simulink model "Ieee14_CC_2019b"  (R2019b)
settings: Solver=ode1  StartTime=0.0  StopTime=3600  FixedStep=1e-3  MaxStep=1e-4  RelTol=1e-3
model workspace (MAT data in the model file):
  pruebaValor = 0
libraries: powerlib x118, dspnetwork x116, source_mod x14, simulink x1
(part 3 of 3)

== system Ieee14_CC_2019b/SM 2 ==
  Constant : Constant  Value=0
  Constant1 : Constant
  Constant2 : Constant  Value=2
  Constant3 : Constant  Value=0
  Constant4 : Constant
  Constant5 : Constant  Value=2
  Index Vector{,1..5} (6 alike) : MultiPortSwitch  DataPortOrder=Zero-based contiguous  Inputs=1  zeroidx=on
  Three-Phase V-I Measurement : powerlib/Measurements/Three-Phase V-I Measurement  VoltageMeasurement=phase-to-ground  SetLabelV=off  LabelV=Vabc  Vpu=on  VpuLL=off  CurrentMeasurement=yes  SetLabelI=off  LabelI=Iabc  Ipu=on  Pbase=100e6  Vbase=69e3  OutputType=Complex  PhasorSimulation=off  PSBequivalent=0
      settings: SourceProductName=Simscape Electrical
  UDP Send Ia : dspnetwork/UDP Send  remoteURL='10.0.255.255'  remotePort=20022  localURL='255.255.255.255'  localPortSource=Automatically determine  localPort=-1  sampletime=-1  blockPlatform=LINUX  separateLengthPort=0
      settings: SourceProductName=Simulink
  UDP Send Ib : dspnetwork/UDP Send  remoteURL='10.0.255.255'  remotePort=20021  localURL='255.255.255.255'  localPortSource=Automatically determine  localPort=-1  sampletime=-1  blockPlatform=LINUX  separateLengthPort=0
      settings: SourceProductName=Simulink
  UDP Send Ic : dspnetwork/UDP Send  remoteURL='10.0.255.255'  remotePort=20020  localURL='255.255.255.255'  localPortSource=Automatically determine  localPort=-1  sampletime=-1  blockPlatform=LINUX  separateLengthPort=0
      settings: SourceProductName=Simulink
  UDP Send Va : dspnetwork/UDP Send  remoteURL='10.0.255.255'  remotePort=10020  localURL='255.255.255.255'  localPortSource=Automatically determine  localPort=-1  sampletime=-1  blockPlatform=LINUX  separateLengthPort=0
      settings: SourceProductName=Simulink
  UDP Send Vb : dspnetwork/UDP Send  remoteURL='10.0.255.255'  remotePort=10021  localURL='255.255.255.255'  localPortSource=Automatically determine  localPort=-1  sampletime=-1  blockPlatform=LINUX  separateLengthPort=0
      settings: SourceProductName=Simulink
  UDP Send Vc : dspnetwork/UDP Send  remoteURL='10.0.255.255'  remotePort=10022  localURL='255.255.255.255'  localPortSource=Automatically determine  localPort=-1  sampletime=-1  blockPlatform=LINUX  separateLengthPort=0
      settings: SourceProductName=Simulink
  a : PMIOPort  Side=Left
  b : PMIOPort  Port=2  Side=Left
  c : PMIOPort  Port=3  Side=Left
  A : PMIOPort  Port=4  Side=Right
  B : PMIOPort  Port=5  Side=Right
  C : PMIOPort  Port=6  Side=Right
  Vabc : Outport
  Iabc : Outport  Port=2
  wires:
  Index Vector/1 -> UDP Send Va/1
  Constant1/1 -> Index Vector1/1
  Constant/1 -> Index Vector/1
  Index Vector2/1 -> UDP Send Vc/1
  Index Vector1/1 -> UDP Send Vb/1
  Constant2/1 -> Index Vector2/1
  Three-Phase V-I Measurement/1 -> Index Vector2/2, Index Vector/2, Index Vector1/2, Vabc/1
  Index Vector4/1 -> UDP Send Ib/1
  Constant3/1 -> Index Vector3/1
  Index Vector3/1 -> UDP Send Ic/1
  Constant5/1 -> Index Vector5/1
  Constant4/1 -> Index Vector4/1
  Index Vector5/1 -> UDP Send Ia/1
  Three-Phase V-I Measurement/2 -> Iabc/1, Index Vector3/2, Index Vector4/2, Index Vector5/2
  connections:
  b/RConn1 -- Three-Phase V-I Measurement/RConn2
  a/RConn1 -- Three-Phase V-I Measurement/RConn1
  c/RConn1 -- Three-Phase V-I Measurement/RConn3
  A/RConn1 -- Three-Phase V-I Measurement/LConn1
  B/RConn1 -- Three-Phase V-I Measurement/LConn2
  C/RConn1 -- Three-Phase V-I Measurement/LConn3

== system Ieee14_CC_2019b/SM 3 ==
  Constant : Constant  Value=0
  Constant1 : Constant
  Constant2 : Constant  Value=2
  Constant3 : Constant  Value=0
  Constant4 : Constant
  Constant5 : Constant  Value=2
  Index Vector{,1..5} (6 alike) : MultiPortSwitch  DataPortOrder=Zero-based contiguous  Inputs=1  zeroidx=on
  Three-Phase V-I Measurement : powerlib/Measurements/Three-Phase V-I Measurement  VoltageMeasurement=phase-to-ground  SetLabelV=off  LabelV=Vabc  Vpu=on  VpuLL=off  CurrentMeasurement=yes  SetLabelI=off  LabelI=Iabc  Ipu=on  Pbase=100e6  Vbase=69e3  OutputType=Complex  PhasorSimulation=off  PSBequivalent=0
      settings: SourceProductName=Simscape Electrical
  UDP Send Ia : dspnetwork/UDP Send  remoteURL='10.0.255.255'  remotePort=20032  localURL='255.255.255.255'  localPortSource=Automatically determine  localPort=-1  sampletime=-1  blockPlatform=LINUX  separateLengthPort=0
      settings: SourceProductName=Simulink
  UDP Send Ib : dspnetwork/UDP Send  remoteURL='10.0.255.255'  remotePort=20031  localURL='255.255.255.255'  localPortSource=Automatically determine  localPort=-1  sampletime=-1  blockPlatform=LINUX  separateLengthPort=0
      settings: SourceProductName=Simulink
  UDP Send Ic : dspnetwork/UDP Send  remoteURL='10.0.255.255'  remotePort=20030  localURL='255.255.255.255'  localPortSource=Automatically determine  localPort=-1  sampletime=-1  blockPlatform=LINUX  separateLengthPort=0
      settings: SourceProductName=Simulink
  UDP Send Va : dspnetwork/UDP Send  remoteURL='10.0.255.255'  remotePort=10030  localURL='255.255.255.255'  localPortSource=Automatically determine  localPort=-1  sampletime=-1  blockPlatform=LINUX  separateLengthPort=0
      settings: SourceProductName=Simulink
  UDP Send Vb : dspnetwork/UDP Send  remoteURL='10.0.255.255'  remotePort=10031  localURL='255.255.255.255'  localPortSource=Automatically determine  localPort=-1  sampletime=-1  blockPlatform=LINUX  separateLengthPort=0
      settings: SourceProductName=Simulink
  UDP Send Vc : dspnetwork/UDP Send  remoteURL='10.0.255.255'  remotePort=10032  localURL='255.255.255.255'  localPortSource=Automatically determine  localPort=-1  sampletime=-1  blockPlatform=LINUX  separateLengthPort=0
      settings: SourceProductName=Simulink
  a : PMIOPort  Side=Left
  b : PMIOPort  Port=2  Side=Left
  c : PMIOPort  Port=3  Side=Left
  A : PMIOPort  Port=4  Side=Right
  B : PMIOPort  Port=5  Side=Right
  C : PMIOPort  Port=6  Side=Right
  Vabc : Outport
  Iabc : Outport  Port=2
  wires:
  Index Vector/1 -> UDP Send Va/1
  Constant1/1 -> Index Vector1/1
  Constant/1 -> Index Vector/1
  Index Vector2/1 -> UDP Send Vc/1
  Index Vector1/1 -> UDP Send Vb/1
  Constant2/1 -> Index Vector2/1
  Three-Phase V-I Measurement/1 -> Index Vector2/2, Index Vector/2, Index Vector1/2, Vabc/1
  Index Vector4/1 -> UDP Send Ib/1
  Constant3/1 -> Index Vector3/1
  Index Vector3/1 -> UDP Send Ic/1
  Constant5/1 -> Index Vector5/1
  Constant4/1 -> Index Vector4/1
  Index Vector5/1 -> UDP Send Ia/1
  Three-Phase V-I Measurement/2 -> Iabc/1, Index Vector3/2, Index Vector4/2, Index Vector5/2
  connections:
  b/RConn1 -- Three-Phase V-I Measurement/RConn2
  a/RConn1 -- Three-Phase V-I Measurement/RConn1
  c/RConn1 -- Three-Phase V-I Measurement/RConn3
  A/RConn1 -- Three-Phase V-I Measurement/LConn1
  B/RConn1 -- Three-Phase V-I Measurement/LConn2
  C/RConn1 -- Three-Phase V-I Measurement/LConn3

== system Ieee14_CC_2019b/SM 4 ==
  Constant : Constant  Value=0
  Constant1 : Constant
  Constant2 : Constant  Value=2
  Constant3 : Constant  Value=0
  Constant4 : Constant
  Constant5 : Constant  Value=2
  Index Vector{,1..5} (6 alike) : MultiPortSwitch  DataPortOrder=Zero-based contiguous  Inputs=1  zeroidx=on
  Three-Phase V-I Measurement : powerlib/Measurements/Three-Phase V-I Measurement  VoltageMeasurement=phase-to-ground  SetLabelV=off  LabelV=Vabc  Vpu=on  VpuLL=off  CurrentMeasurement=yes  SetLabelI=off  LabelI=Iabc  Ipu=on  Pbase=100e6  Vbase=69e3  OutputType=Complex  PhasorSimulation=off  PSBequivalent=0
      settings: SourceProductName=Simscape Electrical
  UDP Send Ia : dspnetwork/UDP Send  remoteURL='10.0.255.255'  remotePort=20042  localURL='255.255.255.255'  localPortSource=Automatically determine  localPort=-1  sampletime=-1  blockPlatform=LINUX  separateLengthPort=0
      settings: SourceProductName=Simulink
  UDP Send Ib : dspnetwork/UDP Send  remoteURL='10.0.255.255'  remotePort=20041  localURL='255.255.255.255'  localPortSource=Automatically determine  localPort=-1  sampletime=-1  blockPlatform=LINUX  separateLengthPort=0
      settings: SourceProductName=Simulink
  UDP Send Ic : dspnetwork/UDP Send  remoteURL='10.0.255.255'  remotePort=20040  localURL='255.255.255.255'  localPortSource=Automatically determine  localPort=-1  sampletime=-1  blockPlatform=LINUX  separateLengthPort=0
      settings: SourceProductName=Simulink
  UDP Send Va : dspnetwork/UDP Send  remoteURL='10.0.255.255'  remotePort=10040  localURL='255.255.255.255'  localPortSource=Automatically determine  localPort=-1  sampletime=-1  blockPlatform=LINUX  separateLengthPort=0
      settings: SourceProductName=Simulink
  UDP Send Vb : dspnetwork/UDP Send  remoteURL='10.0.255.255'  remotePort=10041  localURL='255.255.255.255'  localPortSource=Automatically determine  localPort=-1  sampletime=-1  blockPlatform=LINUX  separateLengthPort=0
      settings: SourceProductName=Simulink
  UDP Send Vc : dspnetwork/UDP Send  remoteURL='10.0.255.255'  remotePort=10042  localURL='255.255.255.255'  localPortSource=Automatically determine  localPort=-1  sampletime=-1  blockPlatform=LINUX  separateLengthPort=0
      settings: SourceProductName=Simulink
  a : PMIOPort  Side=Left
  b : PMIOPort  Port=2  Side=Left
  c : PMIOPort  Port=3  Side=Left
  A : PMIOPort  Port=4  Side=Right
  B : PMIOPort  Port=5  Side=Right
  C : PMIOPort  Port=6  Side=Right
  Vabc : Outport
  Iabc : Outport  Port=2
  wires:
  Index Vector/1 -> UDP Send Va/1
  Constant1/1 -> Index Vector1/1
  Constant/1 -> Index Vector/1
  Index Vector2/1 -> UDP Send Vc/1
  Index Vector1/1 -> UDP Send Vb/1
  Constant2/1 -> Index Vector2/1
  Three-Phase V-I Measurement/1 -> Index Vector2/2, Index Vector/2, Index Vector1/2, Vabc/1
  Index Vector4/1 -> UDP Send Ib/1
  Constant3/1 -> Index Vector3/1
  Index Vector3/1 -> UDP Send Ic/1
  Constant5/1 -> Index Vector5/1
  Constant4/1 -> Index Vector4/1
  Index Vector5/1 -> UDP Send Ia/1
  Three-Phase V-I Measurement/2 -> Iabc/1, Index Vector3/2, Index Vector4/2, Index Vector5/2
  connections:
  b/RConn1 -- Three-Phase V-I Measurement/RConn2
  a/RConn1 -- Three-Phase V-I Measurement/RConn1
  c/RConn1 -- Three-Phase V-I Measurement/RConn3
  A/RConn1 -- Three-Phase V-I Measurement/LConn1
  B/RConn1 -- Three-Phase V-I Measurement/LConn2
  C/RConn1 -- Three-Phase V-I Measurement/LConn3

== system Ieee14_CC_2019b/SM 5 ==
  Constant : Constant  Value=0
  Constant1 : Constant
  Constant2 : Constant  Value=2
  Constant3 : Constant  Value=0
  Constant4 : Constant
  Constant5 : Constant  Value=2
  Index Vector{,1..5} (6 alike) : MultiPortSwitch  DataPortOrder=Zero-based contiguous  Inputs=1  zeroidx=on
  Three-Phase V-I Measurement : powerlib/Measurements/Three-Phase V-I Measurement  VoltageMeasurement=phase-to-ground  SetLabelV=off  LabelV=Vabc  Vpu=on  VpuLL=off  CurrentMeasurement=yes  SetLabelI=off  LabelI=Iabc  Ipu=on  Pbase=100e6  Vbase=69e3  OutputType=Complex  PhasorSimulation=off  PSBequivalent=0
      settings: SourceProductName=Simscape Electrical
  UDP Send Ia : dspnetwork/UDP Send  remoteURL='10.0.255.255'  remotePort=20052  localURL='255.255.255.255'  localPortSource=Automatically determine  localPort=-1  sampletime=-1  blockPlatform=LINUX  separateLengthPort=0
      settings: SourceProductName=Simulink
  UDP Send Ib : dspnetwork/UDP Send  remoteURL='10.0.255.255'  remotePort=20051  localURL='255.255.255.255'  localPortSource=Automatically determine  localPort=-1  sampletime=-1  blockPlatform=LINUX  separateLengthPort=0
      settings: SourceProductName=Simulink
  UDP Send Ic : dspnetwork/UDP Send  remoteURL='10.0.255.255'  remotePort=20050  localURL='255.255.255.255'  localPortSource=Automatically determine  localPort=-1  sampletime=-1  blockPlatform=LINUX  separateLengthPort=0
      settings: SourceProductName=Simulink
  UDP Send Va : dspnetwork/UDP Send  remoteURL='10.0.255.255'  remotePort=10050  localURL='255.255.255.255'  localPortSource=Automatically determine  localPort=-1  sampletime=-1  blockPlatform=LINUX  separateLengthPort=0
      settings: SourceProductName=Simulink
  UDP Send Vb : dspnetwork/UDP Send  remoteURL='10.0.255.255'  remotePort=10051  localURL='255.255.255.255'  localPortSource=Automatically determine  localPort=-1  sampletime=-1  blockPlatform=LINUX  separateLengthPort=0
      settings: SourceProductName=Simulink
  UDP Send Vc : dspnetwork/UDP Send  remoteURL='10.0.255.255'  remotePort=10052  localURL='255.255.255.255'  localPortSource=Automatically determine  localPort=-1  sampletime=-1  blockPlatform=LINUX  separateLengthPort=0
      settings: SourceProductName=Simulink
  a : PMIOPort  Side=Left
  b : PMIOPort  Port=2  Side=Left
  c : PMIOPort  Port=3  Side=Left
  A : PMIOPort  Port=4  Side=Right
  B : PMIOPort  Port=5  Side=Right
  C : PMIOPort  Port=6  Side=Right
  Vabc : Outport
  Iabc : Outport  Port=2
  wires:
  Index Vector/1 -> UDP Send Va/1
  Constant1/1 -> Index Vector1/1
  Constant/1 -> Index Vector/1
  Index Vector2/1 -> UDP Send Vc/1
  Index Vector1/1 -> UDP Send Vb/1
  Constant2/1 -> Index Vector2/1
  Three-Phase V-I Measurement/1 -> Index Vector2/2, Index Vector/2, Index Vector1/2, Vabc/1
  Index Vector4/1 -> UDP Send Ib/1
  Constant3/1 -> Index Vector3/1
  Index Vector3/1 -> UDP Send Ic/1
  Constant5/1 -> Index Vector5/1
  Constant4/1 -> Index Vector4/1
  Index Vector5/1 -> UDP Send Ia/1
  Three-Phase V-I Measurement/2 -> Iabc/1, Index Vector3/2, Index Vector4/2, Index Vector5/2
  connections:
  b/RConn1 -- Three-Phase V-I Measurement/RConn2
  a/RConn1 -- Three-Phase V-I Measurement/RConn1
  c/RConn1 -- Three-Phase V-I Measurement/RConn3
  A/RConn1 -- Three-Phase V-I Measurement/LConn1
  B/RConn1 -- Three-Phase V-I Measurement/LConn2
  C/RConn1 -- Three-Phase V-I Measurement/LConn3

== system Ieee14_CC_2019b/SM 6 ==
  Constant : Constant  Value=0
  Constant1 : Constant
  Constant2 : Constant  Value=2
  Constant3 : Constant  Value=0
  Constant4 : Constant
  Constant5 : Constant  Value=2
  Index Vector{,1..5} (6 alike) : MultiPortSwitch  DataPortOrder=Zero-based contiguous  Inputs=1  zeroidx=on
  Three-Phase V-I Measurement : powerlib/Measurements/Three-Phase V-I Measurement  VoltageMeasurement=phase-to-ground  SetLabelV=off  LabelV=Vabc  Vpu=on  VpuLL=off  CurrentMeasurement=yes  SetLabelI=off  LabelI=Iabc  Ipu=on  Pbase=100e6  Vbase=69e3  OutputType=Complex  PhasorSimulation=off  PSBequivalent=0
      settings: SourceProductName=Simscape Electrical
  UDP Send Ia : dspnetwork/UDP Send  remoteURL='10.0.255.255'  remotePort=20062  localURL='255.255.255.255'  localPortSource=Automatically determine  localPort=-1  sampletime=-1  blockPlatform=LINUX  separateLengthPort=0
      settings: SourceProductName=Simulink
  UDP Send Ib : dspnetwork/UDP Send  remoteURL='10.0.255.255'  remotePort=20061  localURL='255.255.255.255'  localPortSource=Automatically determine  localPort=-1  sampletime=-1  blockPlatform=LINUX  separateLengthPort=0
      settings: SourceProductName=Simulink
  UDP Send Ic : dspnetwork/UDP Send  remoteURL='10.0.255.255'  remotePort=20060  localURL='255.255.255.255'  localPortSource=Automatically determine  localPort=-1  sampletime=-1  blockPlatform=LINUX  separateLengthPort=0
      settings: SourceProductName=Simulink
  UDP Send Va : dspnetwork/UDP Send  remoteURL='10.0.255.255'  remotePort=10060  localURL='255.255.255.255'  localPortSource=Automatically determine  localPort=-1  sampletime=-1  blockPlatform=LINUX  separateLengthPort=0
      settings: SourceProductName=Simulink
  UDP Send Vb : dspnetwork/UDP Send  remoteURL='10.0.255.255'  remotePort=10061  localURL='255.255.255.255'  localPortSource=Automatically determine  localPort=-1  sampletime=-1  blockPlatform=LINUX  separateLengthPort=0
      settings: SourceProductName=Simulink
  UDP Send Vc : dspnetwork/UDP Send  remoteURL='10.0.255.255'  remotePort=10062  localURL='255.255.255.255'  localPortSource=Automatically determine  localPort=-1  sampletime=-1  blockPlatform=LINUX  separateLengthPort=0
      settings: SourceProductName=Simulink
  a : PMIOPort  Side=Left
  b : PMIOPort  Port=2  Side=Left
  c : PMIOPort  Port=3  Side=Left
  A : PMIOPort  Port=4  Side=Right
  B : PMIOPort  Port=5  Side=Right
  C : PMIOPort  Port=6  Side=Right
  Vabc : Outport
  Iabc : Outport  Port=2
  wires:
  Index Vector/1 -> UDP Send Va/1
  Constant1/1 -> Index Vector1/1
  Constant/1 -> Index Vector/1
  Index Vector2/1 -> UDP Send Vc/1
  Index Vector1/1 -> UDP Send Vb/1
  Constant2/1 -> Index Vector2/1
  Three-Phase V-I Measurement/1 -> Index Vector2/2, Index Vector/2, Index Vector1/2, Vabc/1
  Index Vector4/1 -> UDP Send Ib/1
  Constant3/1 -> Index Vector3/1
  Index Vector3/1 -> UDP Send Ic/1
  Constant5/1 -> Index Vector5/1
  Constant4/1 -> Index Vector4/1
  Index Vector5/1 -> UDP Send Ia/1
  Three-Phase V-I Measurement/2 -> Iabc/1, Index Vector3/2, Index Vector4/2, Index Vector5/2
  connections:
  b/RConn1 -- Three-Phase V-I Measurement/RConn2
  a/RConn1 -- Three-Phase V-I Measurement/RConn1
  c/RConn1 -- Three-Phase V-I Measurement/RConn3
  A/RConn1 -- Three-Phase V-I Measurement/LConn1
  B/RConn1 -- Three-Phase V-I Measurement/LConn2
  C/RConn1 -- Three-Phase V-I Measurement/LConn3

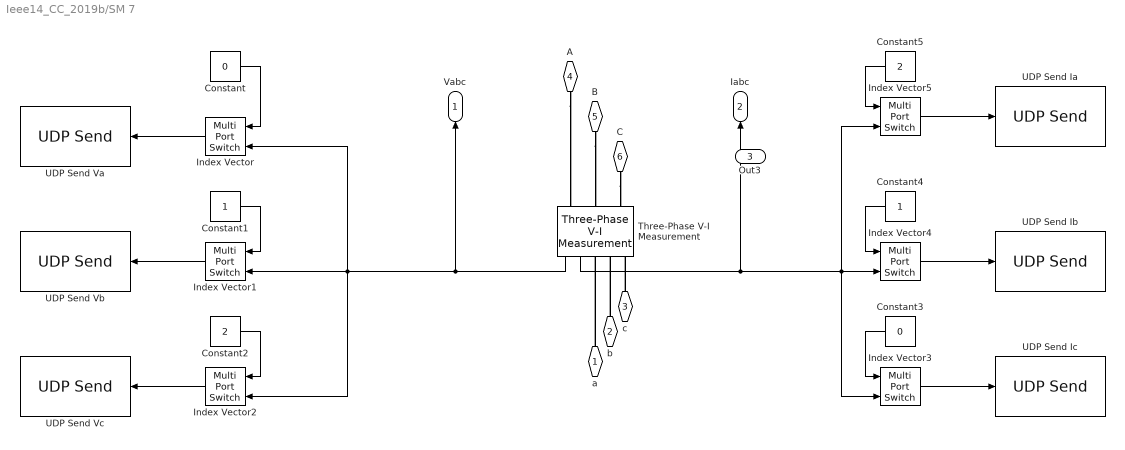
== system Ieee14_CC_2019b/SM 7 ==
  Constant : Constant  Value=0
  Constant1 : Constant
  Constant2 : Constant  Value=2
  Constant3 : Constant  Value=0
  Constant4 : Constant
  Constant5 : Constant  Value=2
  Index Vector{,1..5} (6 alike) : MultiPortSwitch  DataPortOrder=Zero-based contiguous  Inputs=1  zeroidx=on
  Three-Phase V-I Measurement : powerlib/Measurements/Three-Phase V-I Measurement  VoltageMeasurement=phase-to-ground  SetLabelV=off  LabelV=Vabc  Vpu=on  VpuLL=off  CurrentMeasurement=yes  SetLabelI=off  LabelI=Iabc  Ipu=on  Pbase=100e6  Vbase=69e3  OutputType=Complex  PhasorSimulation=off  PSBequivalent=0
      settings: SourceProductName=Simscape Electrical
  UDP Send Ia : dspnetwork/UDP Send  remoteURL='10.0.255.255'  remotePort=20072  localURL='255.255.255.255'  localPortSource=Automatically determine  localPort=-1  sampletime=-1  blockPlatform=LINUX  separateLengthPort=0
      settings: SourceProductName=Simulink
  UDP Send Ib : dspnetwork/UDP Send  remoteURL='10.0.255.255'  remotePort=20071  localURL='255.255.255.255'  localPortSource=Automatically determine  localPort=-1  sampletime=-1  blockPlatform=LINUX  separateLengthPort=0
      settings: SourceProductName=Simulink
  UDP Send Ic : dspnetwork/UDP Send  remoteURL='10.0.255.255'  remotePort=20070  localURL='255.255.255.255'  localPortSource=Automatically determine  localPort=-1  sampletime=-1  blockPlatform=LINUX  separateLengthPort=0
      settings: SourceProductName=Simulink
  UDP Send Va : dspnetwork/UDP Send  remoteURL='10.0.255.255'  remotePort=10070  localURL='255.255.255.255'  localPortSource=Automatically determine  localPort=-1  sampletime=-1  blockPlatform=LINUX  separateLengthPort=0
      settings: SourceProductName=Simulink
  UDP Send Vb : dspnetwork/UDP Send  remoteURL='10.0.255.255'  remotePort=10071  localURL='255.255.255.255'  localPortSource=Automatically determine  localPort=-1  sampletime=-1  blockPlatform=LINUX  separateLengthPort=0
      settings: SourceProductName=Simulink
  UDP Send Vc : dspnetwork/UDP Send  remoteURL='10.0.255.255'  remotePort=10072  localURL='255.255.255.255'  localPortSource=Automatically determine  localPort=-1  sampletime=-1  blockPlatform=LINUX  separateLengthPort=0
      settings: SourceProductName=Simulink
  a : PMIOPort  Side=Left
  b : PMIOPort  Port=2  Side=Left
  c : PMIOPort  Port=3  Side=Left
  A : PMIOPort  Port=4  Side=Right
  B : PMIOPort  Port=5  Side=Right
  C : PMIOPort  Port=6  Side=Right
  Vabc : Outport
  Iabc : Outport  Port=2
  Out3 : Outport  Port=3
  wires:
  Index Vector/1 -> UDP Send Va/1
  Constant1/1 -> Index Vector1/1
  Constant/1 -> Index Vector/1
  Index Vector2/1 -> UDP Send Vc/1
  Index Vector1/1 -> UDP Send Vb/1
  Constant2/1 -> Index Vector2/1
  Three-Phase V-I Measurement/1 -> Index Vector2/2, Index Vector/2, Index Vector1/2, Vabc/1
  Index Vector4/1 -> UDP Send Ib/1
  Constant3/1 -> Index Vector3/1
  Index Vector3/1 -> UDP Send Ic/1
  Constant5/1 -> Index Vector5/1
  Constant4/1 -> Index Vector4/1
  Index Vector5/1 -> UDP Send Ia/1
  Three-Phase V-I Measurement/2 -> Iabc/1, Index Vector3/2, Index Vector4/2, Index Vector5/2
  connections:
  b/RConn1 -- Three-Phase V-I Measurement/RConn2
  a/RConn1 -- Three-Phase V-I Measurement/RConn1
  c/RConn1 -- Three-Phase V-I Measurement/RConn3
  A/RConn1 -- Three-Phase V-I Measurement/LConn1
  B/RConn1 -- Three-Phase V-I Measurement/LConn2
  C/RConn1 -- Three-Phase V-I Measurement/LConn3

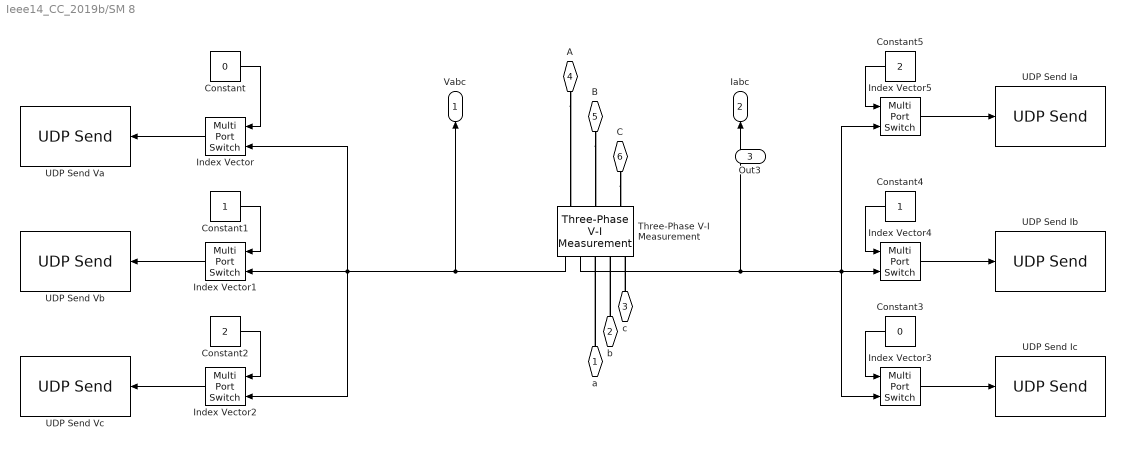
== system Ieee14_CC_2019b/SM 8 ==
  Constant : Constant  Value=0
  Constant1 : Constant
  Constant2 : Constant  Value=2
  Constant3 : Constant  Value=0
  Constant4 : Constant
  Constant5 : Constant  Value=2
  Index Vector{,1..5} (6 alike) : MultiPortSwitch  DataPortOrder=Zero-based contiguous  Inputs=1  zeroidx=on
  Three-Phase V-I Measurement : powerlib/Measurements/Three-Phase V-I Measurement  VoltageMeasurement=phase-to-ground  SetLabelV=off  LabelV=Vabc  Vpu=on  VpuLL=off  CurrentMeasurement=yes  SetLabelI=off  LabelI=Iabc  Ipu=on  Pbase=100e6  Vbase=69e3  OutputType=Complex  PhasorSimulation=off  PSBequivalent=0
      settings: SourceProductName=Simscape Electrical
  UDP Send Ia : dspnetwork/UDP Send  remoteURL='10.0.255.255'  remotePort=20082  localURL='255.255.255.255'  localPortSource=Automatically determine  localPort=-1  sampletime=-1  blockPlatform=LINUX  separateLengthPort=0
      settings: SourceProductName=Simulink
  UDP Send Ib : dspnetwork/UDP Send  remoteURL='10.0.255.255'  remotePort=20081  localURL='255.255.255.255'  localPortSource=Automatically determine  localPort=-1  sampletime=-1  blockPlatform=LINUX  separateLengthPort=0
      settings: SourceProductName=Simulink
  UDP Send Ic : dspnetwork/UDP Send  remoteURL='10.0.255.255'  remotePort=20080  localURL='255.255.255.255'  localPortSource=Automatically determine  localPort=-1  sampletime=-1  blockPlatform=LINUX  separateLengthPort=0
      settings: SourceProductName=Simulink
  UDP Send Va : dspnetwork/UDP Send  remoteURL='10.0.255.255'  remotePort=10080  localURL='255.255.255.255'  localPortSource=Automatically determine  localPort=-1  sampletime=-1  blockPlatform=LINUX  separateLengthPort=0
      settings: SourceProductName=Simulink
  UDP Send Vb : dspnetwork/UDP Send  remoteURL='10.0.255.255'  remotePort=10081  localURL='255.255.255.255'  localPortSource=Automatically determine  localPort=-1  sampletime=-1  blockPlatform=LINUX  separateLengthPort=0
      settings: SourceProductName=Simulink
  UDP Send Vc : dspnetwork/UDP Send  remoteURL='10.0.255.255'  remotePort=10082  localURL='255.255.255.255'  localPortSource=Automatically determine  localPort=-1  sampletime=-1  blockPlatform=LINUX  separateLengthPort=0
      settings: SourceProductName=Simulink
  a : PMIOPort  Side=Left
  b : PMIOPort  Port=2  Side=Left
  c : PMIOPort  Port=3  Side=Left
  A : PMIOPort  Port=4  Side=Right
  B : PMIOPort  Port=5  Side=Right
  C : PMIOPort  Port=6  Side=Right
  Vabc : Outport
  Iabc : Outport  Port=2
  Out3 : Outport  Port=3
  wires:
  Index Vector/1 -> UDP Send Va/1
  Constant1/1 -> Index Vector1/1
  Constant/1 -> Index Vector/1
  Index Vector2/1 -> UDP Send Vc/1
  Index Vector1/1 -> UDP Send Vb/1
  Constant2/1 -> Index Vector2/1
  Three-Phase V-I Measurement/1 -> Index Vector2/2, Index Vector/2, Index Vector1/2, Vabc/1
  Index Vector4/1 -> UDP Send Ib/1
  Constant3/1 -> Index Vector3/1
  Index Vector3/1 -> UDP Send Ic/1
  Constant5/1 -> Index Vector5/1
  Constant4/1 -> Index Vector4/1
  Index Vector5/1 -> UDP Send Ia/1
  Three-Phase V-I Measurement/2 -> Iabc/1, Index Vector3/2, Index Vector4/2, Index Vector5/2
  connections:
  b/RConn1 -- Three-Phase V-I Measurement/RConn2
  a/RConn1 -- Three-Phase V-I Measurement/RConn1
  c/RConn1 -- Three-Phase V-I Measurement/RConn3
  A/RConn1 -- Three-Phase V-I Measurement/LConn1
  B/RConn1 -- Three-Phase V-I Measurement/LConn2
  C/RConn1 -- Three-Phase V-I Measurement/LConn3

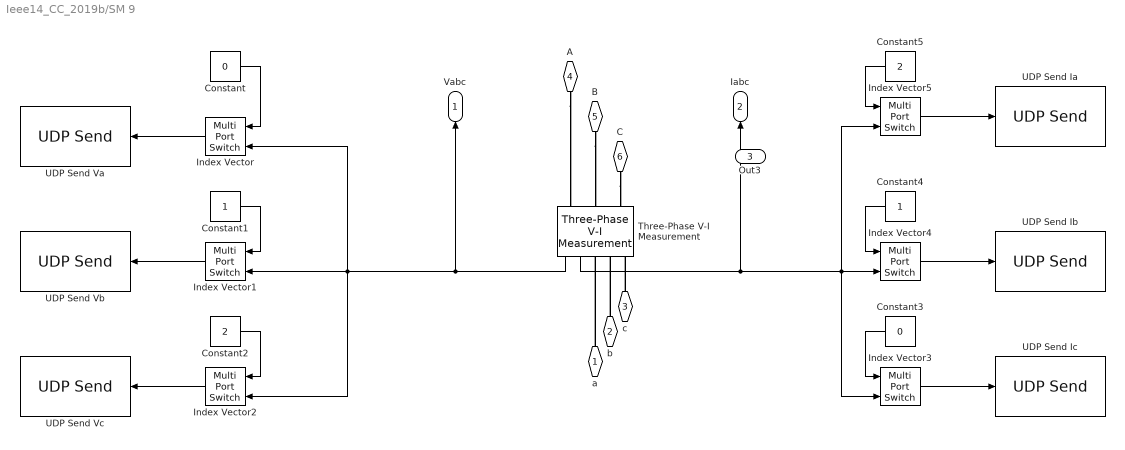
== system Ieee14_CC_2019b/SM 9 ==
  Constant : Constant  Value=0
  Constant1 : Constant
  Constant2 : Constant  Value=2
  Constant3 : Constant  Value=0
  Constant4 : Constant
  Constant5 : Constant  Value=2
  Index Vector{,1..5} (6 alike) : MultiPortSwitch  DataPortOrder=Zero-based contiguous  Inputs=1  zeroidx=on
  Three-Phase V-I Measurement : powerlib/Measurements/Three-Phase V-I Measurement  VoltageMeasurement=phase-to-ground  SetLabelV=off  LabelV=Vabc  Vpu=on  VpuLL=off  CurrentMeasurement=yes  SetLabelI=off  LabelI=Iabc  Ipu=on  Pbase=100e6  Vbase=69e3  OutputType=Complex  PhasorSimulation=off  PSBequivalent=0
      settings: SourceProductName=Simscape Electrical
  UDP Send Ia : dspnetwork/UDP Send  remoteURL='10.0.255.255'  remotePort=20092  localURL='255.255.255.255'  localPortSource=Automatically determine  localPort=-1  sampletime=-1  blockPlatform=LINUX  separateLengthPort=0
      settings: SourceProductName=Simulink
  UDP Send Ib : dspnetwork/UDP Send  remoteURL='10.0.255.255'  remotePort=20091  localURL='255.255.255.255'  localPortSource=Automatically determine  localPort=-1  sampletime=-1  blockPlatform=LINUX  separateLengthPort=0
      settings: SourceProductName=Simulink
  UDP Send Ic : dspnetwork/UDP Send  remoteURL='10.0.255.255'  remotePort=20090  localURL='255.255.255.255'  localPortSource=Automatically determine  localPort=-1  sampletime=-1  blockPlatform=LINUX  separateLengthPort=0
      settings: SourceProductName=Simulink
  UDP Send Va : dspnetwork/UDP Send  remoteURL='10.0.255.255'  remotePort=10090  localURL='255.255.255.255'  localPortSource=Automatically determine  localPort=-1  sampletime=-1  blockPlatform=LINUX  separateLengthPort=0
      settings: SourceProductName=Simulink
  UDP Send Vb : dspnetwork/UDP Send  remoteURL='10.0.255.255'  remotePort=10091  localURL='255.255.255.255'  localPortSource=Automatically determine  localPort=-1  sampletime=-1  blockPlatform=LINUX  separateLengthPort=0
      settings: SourceProductName=Simulink
  UDP Send Vc : dspnetwork/UDP Send  remoteURL='10.0.255.255'  remotePort=10092  localURL='255.255.255.255'  localPortSource=Automatically determine  localPort=-1  sampletime=-1  blockPlatform=LINUX  separateLengthPort=0
      settings: SourceProductName=Simulink
  a : PMIOPort  Side=Left
  b : PMIOPort  Port=2  Side=Left
  c : PMIOPort  Port=3  Side=Left
  A : PMIOPort  Port=4  Side=Right
  B : PMIOPort  Port=5  Side=Right
  C : PMIOPort  Port=6  Side=Right
  Vabc : Outport
  Iabc : Outport  Port=2
  Out3 : Outport  Port=3
  wires:
  Index Vector/1 -> UDP Send Va/1
  Constant1/1 -> Index Vector1/1
  Constant/1 -> Index Vector/1
  Index Vector2/1 -> UDP Send Vc/1
  Index Vector1/1 -> UDP Send Vb/1
  Constant2/1 -> Index Vector2/1
  Three-Phase V-I Measurement/1 -> Index Vector2/2, Index Vector/2, Index Vector1/2, Vabc/1
  Index Vector4/1 -> UDP Send Ib/1
  Constant3/1 -> Index Vector3/1
  Index Vector3/1 -> UDP Send Ic/1
  Constant5/1 -> Index Vector5/1
  Constant4/1 -> Index Vector4/1
  Index Vector5/1 -> UDP Send Ia/1
  Three-Phase V-I Measurement/2 -> Iabc/1, Index Vector3/2, Index Vector4/2, Index Vector5/2
  connections:
  b/RConn1 -- Three-Phase V-I Measurement/RConn2
  a/RConn1 -- Three-Phase V-I Measurement/RConn1
  c/RConn1 -- Three-Phase V-I Measurement/RConn3
  A/RConn1 -- Three-Phase V-I Measurement/LConn1
  B/RConn1 -- Three-Phase V-I Measurement/LConn2
  C/RConn1 -- Three-Phase V-I Measurement/LConn3

== matlab function Ieee14_CC_2019b/CC ==
  settings: updateMethod=DISCRETE  sampleTime=10
function fcn()

    %{
    
    Function CC: short circuits.
    
    Details: This function is responsible for causing short circuits throughout the simulation.
    
    Important: In edit Data, you must adjust the time interval for entering this function. If the interval is set to 5 seconds, its behavior is:
    
    T = 5s --> A random fault is activated
    T = 10s --> The fault is deactivated
    T = 15s --> A random fault is activated
    T = 20s --> The fault is deactivated
    ... ... ...
    
    %}

    
    % - - - - - - - - - - - - - - - - - - - - - - - - -
    
    % coders
    coder.extrinsic('mat2str');
    coder.extrinsic('set_param');
    
    % - - - - - - - - - - - - - - - - - - - - - - - - -
    
    % If skip=1, no fault is activated
    skip = 1;
    
    % - - - - - - - - - - - - - - - - - - - - - - - - -
    
    % = = = = = = = = = = = = = = = = = = = = = = = = =
    % = = = = = = = = = = = = = = = = = = = = = = = = =
    % - - - - - - - - Code - - - - - - - - - - - - - 
    % = = = = = = = = = = = = = = = = = = = = = = = = =
    % = = = = = = = = = = = = = = = = = = = = = = = = =
    
    % - - - - - - - - - - - - - - - - - - - - - - - - -
    
    % Activate or skip fault generation
    if skip == 1
        return
    end
    
    % - - - - - - - - - - - - - - - - - - - - - - - - -
    
    % Persisten variables
    
    % attack: if 1, fault is activated (cc)
    persistent fault_active
    if isempty(fault_active)
       fault_active = 0;
       return
    end
    
    % lineCC: line with active fault
    persistent lineCC;
    if isempty(lineCC)
        lineCC = 0;
    end
    
    % - - - - - - - - - - - - - - - - - - - - - - - - -
    
    % Model path
    path = "Ieee14_CC/";
    
    % - - - - - - - - - - - - - - - - - - - - - - - - -
    
    % Restore ataque
    if fault_active == 1
        if lineCC == 0
            line = "L0";
            aux = path + "CC_" + line;
            set_param(aux, 'Value', mat2str(0));
        end
        if lineCC == 1
            line = "L1";
            aux = path + "CC_" + line;
            set_param(aux, 'Value', mat2str(0));
        end
        if lineCC == 2
            line = "L2";
            aux = path + "CC_" + line;
            set_param(aux, 'Value', mat2str(0));
        end
        if lineCC == 3
            line = "L3";
            aux = path + "CC_" + line;
            set_param(aux, 'Value', mat2str(0));
        end
        if lineCC == 4
            line = "L4";
            aux = path + "CC_" + line;
            set_param(aux, 'Value', mat2str(0));
        end
        if lineCC == 5
            line = "L5";
            aux = path + "CC_" + line;
            set_param(aux, 'Value', mat2str(0));
        end
        if lineCC == 6
            line = "L6";
            aux = path + "CC_" + line;
            set_param(aux, 'Value', mat2str(0));
        end
        if lineCC == 7
            line = "L7";
            aux = path + "CC_" + line;
            set_param(aux, 'Value', mat2str(0));
        end
        if lineCC == 8
            line = "L8";
            aux = path + "CC_" + line;
            set_param(aux, 'Value', mat2str(0));
        end
        if lineCC == 9
            line = "L9";
            aux = path + "CC_" + line;
            set_param(aux, 'Value', mat2str(0));
        end
        if lineCC == 10
            line = "L10";
            aux = path + "CC_" + line;
            set_param(aux, 'Value', mat2str(0));
        end
        if lineCC == 11
            line = "L11";
            aux = path + "CC_" + line;
            set_param(aux, 'Value', mat2str(0));
        end
        if lineCC == 12
            line = "L12";
            aux = path + "CC_" + line;
            set_param(aux, 'Value', mat2str(0));
        end
        if lineCC == 13
            line = "L13";
            aux = path + "CC_" + line;
            set_param(aux, 'Value', mat2str(0));
        end
        if lineCC == 14
            line = "L14";
            aux = path + "CC_" + line;
            set_param(aux, 'Value', mat2str(0));
        end
        if lineCC == 15
            line = "L15";
            aux = path + "CC_" + line;
            set_param(aux, 'Value', mat2str(0));
        end
    
        fault_active = 0;
        disp('=============')
        disp('Disconnection CC');
        disp('=============');
        return
    end
    
    % Activate fault

    % Probability of 10% of line failing
    activate = randi(10);
    
    if fault_active == 0 && activate
        % Randomly select line (0-15)
        lineCC = randi(16) - 1;
        disp('=======================');
        disp('=======================');
        disp('LineaCC');
        disp(lineCC);
        disp('=======================');
        disp('=======================');
        if lineCC == 0
            line = "L0";
            aux = path + "CC_" + line;
            set_param(aux, 'Value', mat2str(1));
        end
        if lineCC == 1
            line = "L1";
            aux = path + "CC_" + line;
            set_param(aux, 'Value', mat2str(1));
        end
        if lineCC == 2
            line = "L2";
            aux = path + "CC_" + line;
            set_param(aux, 'Value', mat2str(1));
        end
        if lineCC == 3
            line = "L3";
            aux = path + "CC_" + line;
            set_param(aux, 'Value', mat2str(1));
        end
        if lineCC == 4
            line = "L4";
            aux = path + "CC_" + line;
            set_param(aux, 'Value', mat2str(1));
        end
        if lineCC == 5
            line = "L5";
            aux = path + "CC_" + line;
            set_param(aux, 'Value', mat2str(1));
        end
        if lineCC == 6
            line = "L6";
            aux = path + "CC_" + line;
            set_param(aux, 'Value', mat2str(1));
        end
        if lineCC == 7
            line = "L7";
            aux = path + "CC_" + line;
            set_param(aux, 'Value', mat2str(1));
        end
        if lineCC == 8
            line = "L8";
            aux = path + "CC_" + line;
            set_param(aux, 'Value', mat2str(1));
        end
        if lineCC == 9
            line = "L9";
            aux = path + "CC_" + line;
            set_param(aux, 'Value', mat2str(1));
        end
        if lineCC == 10
            line = "L10";
            aux = path + "CC_" + line;
            set_param(aux, 'Value', mat2str(1));
        end
        if lineCC == 11
            line = "L11";
            aux = path + "CC_" + line;
            set_param(aux, 'Value', mat2str(1));
        end
        if lineCC == 12
            line = "L12";
            aux = path + "CC_" + line;
            set_param(aux, 'Value', mat2str(1));
        end
        if lineCC == 13
            line = "L13";
            aux = path + "CC_" + line;
            set_param(aux, 'Value', mat2str(1));
        end
        if lineCC == 14
            line = "L14";
            aux = path + "CC_" + line;
            set_param(aux, 'Value', mat2str(1));
        end
        if lineCC == 15
            line = "L15";
            aux = path + "CC_" + line;
            set_param(aux, 'Value', mat2str(1));
        end
        fault_active = 1;
        return
    end

end

== matlab function Ieee14_CC_2019b/V_Corrientes ==
  data: u input; t input; total output; status input
function total  = fcn(u,t,status) % poner status

%{

Funcion: V_Corrientes.

Detalles: Este bloque se encarga de preparar las corrientes a partir de 0.2
segundos de simulacion y con el periodo de la señal. No se volvera a
ejecutar hasta que el algoritmo de deteccion permita escuchar a traves del
valor de status. 

Return: Se envia un vector vacio cuando no se tiene los valores calculados,
o se envia un vector con los maximos hasta que el status sea 1 y se pueda
calcular un nuevo periodo de señal.

%}

% - - - - - - - - - - - - - - - - - - - - - - - - - - - 

% Constantes
periodo = 0.02;
tiempoSegu = 0.2;

numValores = (periodo / 0.001) + 1;
numMedidas = size(u,1);

% - - - - - - - - - - - - - - - - - - - - - - - - - - - 

% Persistent

% dataset: guarda los valores de la corriente
persistent dataset;
if isempty(dataset)
    dataset = zeros(numValores,numMedidas);
end

% row: indicar la fila para guardar valores
persistent row;
if isempty(row)
    row = 1;
end

% timeCut: indicar tiempo en el que se deja de guardar valores
persistent timeCut;
if isempty(timeCut)
    timeCut = tiempoSegu + periodo;
end

% openWindow: tiempo en el que se empieza a guardar valores
persistent openWindow;
if isempty(openWindow)
    openWindow = tiempoSegu;
end

% cambio: control de status
persistent cambio;
if isempty(cambio)
    cambio = 0;
end

% - - - - - - - - - - - - - - - - - - - - - - - - - - - 

% Si cambio es 0, forzar status a 0.
if cambio == 0
    status = 0;
end

% - - - - - - - - - - - - - - - - - - - - - - - - - - - 

% Vector vacio, sin medida
vacio = zeros(1,numMedidas);

% - - - - - - - - - - - - - - - - - - - - - - - - - - - 

% Condiciones

% No guarda si t es menor que openWindow
if t < openWindow 
    total = vacio; 
    return;
end

% Se calcula y se envia si t es superior a timeCut
if t > timeCut
    
    % Cambio = 1, status es controlado por el algoritmo y no por cambio.
    cambio = 1;
    
    % Calcular max
    datos = max(dataset);
    
    % Resetear valores
    dataset(1:numValores,1:numMedidas) = 0;
    row = 1;
    
    % Condiciones de cambio
    if status == 1
        openWindow = t;
        timeCut = t + 1e-3 + periodo;
        cambio = 0;
    end
    
    % Enviar datos
    total = datos; 
    return;
end

% - - - - - - - - - - - - - - - - - - - - - - - - - - - 

% Guardar valores si no cumple condiciones anteriores
vector = zeros(1,numMedidas);

for i = 1:numMedidas
    vector(1,i) = u(i); 
end

dataset(row,1:numMedidas) = vector;
row = row + 1;
total = vacio; 
end

== matlab function Ieee14_CC_2019b/InicioFcn ==
  settings: sampleTime=0
  data: u input
function fcn(u)

%{

Funcion: inicioFcn

Detalles: Funcion de inicializacion de la red. Se ejecuta 1 sola vez. 
Llama a la funcion resetRed externa que inicializa los valores de la red.

Adicional: Para evitar cualquier mensaje de warning, se anulan desde la
linea warning('off','all'). A pesar del warning, no es un problema para el
funcionamiento de la red

%}

% - - - - - - - - - - - - - - - - - - - - - - - - -

% Coder
coder.extrinsic('resetRed');
coder.extrinsic('warning');

% - - - - - - - - - - - - - - - - - - - - - - - - -

% Resetar
if u == 0
    resetRed();
    warning('off','all');
end

% - - - - - - - - - - - - - - - - - - - - - - - - -
end

== matlab function Ieee14_CC_2019b/ ajustVBreakers ==
  settings: sampleTime=0.1
  data: estado input; linea input; u input; ordenes output
function ordenes=fcn(estado,linea,u)

%{

Funcin: ajustVBreakers

Detalles: esta funcion se encarga de modificar los valores de los breakers
en funcion del estado predicho. Por ejemplo, si hay una linea con un ataque
de apertura y se envia a abrir, aqui no se aceptara el cambio debido a que
es un ataque y se mantendra cerrado. 

%}

% - - - - - - - - - - - - - - - - - - - - - - - - - - - 

% Coder
coder.extrinsic('mat2str');
coder.extrinsic('set_param');
coder.extrinsic('gcb');
coder.extrinsic('strfind');
coder.extrinsic('reverse');

% - - - - - - - - - - - - - - - - - - - - - - - - - - - 

% Variables de ajuste
% Si esta variable es 1, se aplican los cambios en funcion del estado
% predicho por el algoritmo, si no, es como si el algoritmo no funcionara.
activarAjustVBreakers = 1;

% - - - - - - - - - - - - - - - - - - - - - - - - - - - 

% Persistents

% estActual: guarda el estado actual de los breakers. Default: todos los
% breakers estan cerrados, todos = 1.
persistent estActual;
if isempty(estActual)
    estActual = ones(1,16);
end

% Emergencia por CC
persistent emergenciaFlag;
if isempty(emergenciaFlag)
    emergenciaFlag = false;
end

persistent emergencia;
if isempty(emergencia)
    emergencia = 0;
end

% - - - - - - - - - - - - - - - - - - - - - - - - - - - 

% Direccion
% a = gcb;
% b = reverse(a);
% c = strfind(b,'/');
% b = b(c(1):end);
% direccion = reverse(b);

% Direccion
direccion = "Ieee14_CC/";

% Condiciones

% Si se recibe estado 99, y linea 99, es que no se ha recibido informacion
% y se mantiene igual. 

% if estado == 99  && linea==99
%     Bloque status = 0. 
%     aux = direccion + "c_Status";
%     set_param(aux,'Value',mat2str(0));
%     ordenes = estActual;
%     return
% end

% - - - - - - - - - - - - - - - - - - - - - - - - - - - 

% Si se recibe un estado, siendo 0,1,2,3 o 4: 

% - - - - - - - - - - - - - - - - - - - - - - - - - - - 

% Cambiar vector de interrupciones en funcion del ataque

if activarAjustVBreakers == 1

    if estado == 2 || estado == 3
        valor = u(linea);
        if valor == 0
            valor = 1;
        else
            valor = 0;
        end
        u(linea) = valor;
    end

    % - - - - - - - - - - - - - - - - - - - - - - - - - - - 
    
    % estado = 1, CC
    if estado == 1
        emergenciaFlag = true;
        emergencia = linea;
        u(linea) = 0;
    end

    % Si se detecta estado 0, y esta el flag de emergencia, se regresa a un
    % estado normal.
    if emergenciaFlag == true
        % estado normal
        if estado == 0
            u(emergencia) = 1;
            emergenciaFlag = false;
        else
            u(emergencia) = 0;
        end
    end
end

% - - - - - - - - - - - - - - - - - - - - - - - - - - - 

% Se guarda el estado actual de los breakers y se coloca status = 1 para
% recibir otra serie de datos.
ordenes = u;
estActual = u;
aux = direccion + "c_Status";
set_param(aux,'Value',mat2str(1));
disp('---------------------');
return

end

== matlab function Ieee14_CC_2019b/Algoritmo de deteccion  ==
  data: u input; estado output; vBreakers input; linea output; vBreakers output; status input; corrientesLineas output
function [estado,linea,vBreakers,corrientesLineas]=fcn(u,vBreakers,status)

%{

Funcion: Algoritmo de deteccion

Detalles: Se encarga de recoger el dataset con los valores de los breakers
recibidos a traves del socket, y procesarlo con los modelos entrnados a
traves de la funcion externa << predecir >>. 

Return: la funcion externa devolvera:

    - estado: estado de la red. 0 -> normal, 1-> CC, 2-> medida, ...
    - linea: linea afectada.
    - vBreakers: se envia vBreakers de la entrada
    - corrientesLineas: corrientes que se envian a OMNet++

%}

% - - - - - - - - - - - - - - - - - - - - - - - - - - - 

% Coders
coder.extrinsic('predecir');
coder.extrinsic('get_param');

% - - - - - - - - - - - - - - - - - - - - - - - - - - - 

% Persistent

% operativo: Si es 1, el algoritmo no se ejecuta y espera.
persistent operativo;
if isempty(operativo)
    operativo = 0;
end

% corrientes: guarda los valores de corrientes
persistent corrientes;
if isempty(corrientes)
    corrientes = zeros(size(u));
end

% - - - - - - - - - - - - - - - - - - - - - - - - - - - 

% No calcular si se recibe un vector de corrientes vacio
if sum(u) < 1 && operativo == 0
    estado = 99;
    linea=99;
    corrientesLineas = zeros(1,16);
    return
elseif (operativo == 0) % se almacena las corrientes recibidas
    disp('Actualiza Corrientes')
    corrientes = u;
end

 
% - - - - - - - - - - - - - - - - - - - - - - - - - - - 

operativo = 1;

% Si el status del sistema es 0, se debe esperar.
if status == 0
    estado = 99;
    linea=99;
    corrientesLineas = corrientes(1,1:16);
    return
end

% - - - - - - - - - - - - - - - - - - - - - - - - - - - 

% Se utiliza la configuracion por defecto de la red con las potencias
% predeterminadas de la funcion resetRed y se mezcla con los valores de
% corrientes y los valores de los breakers.

operativo = 0;

% Valores constantes
dataset = [125303101.728227	9671973.1671217	24620000	23943503.6599636 ...
    26220000	-6996015.08852567	0	40917643.0680923	0	...
    17934585.6176152	0	0	15624000	9144000	12388530 ...
    7250430	19091660	11173460	11297020	6611620	12162850	...
    7118350	0	0	0	0	16214240	9489440	17566150	10280650 ...
    18861640	11038840	15079330	8825230	15979880	9352280	16157820 ...
    9456420	1.06	0	1.045	-2.31887803690131	1.02354	-3.2741816196953 ...
    1.01301125373814	-5.72848350928936	1.01424448398754 ...
    -5.4223615574842	1.07	-12.6500089091098	1.05605772029689 ...
    -9.58948853876113	1.08517	-9.58948853876097	1.05041154732629 ...
    -11.5912508273395	1.03587144188204	-12.5245972673176 ...
    1.03392872015978	-13.2816229985229	1.03331569947612 ...
    -13.7642034766448	1.03892582086589	-13.5133804516998	... 
    1.01960089822285	-13.3762713279553];

% Valores de potencia + tensiones + corrientes + vBreakers
dataset = [dataset corrientes vBreakers];

% Ejecutar modelos y predecir estado y linea
[estado,linea] = predecir(dataset);

% En caso de ejecucion, se envia un vector vacio a OMNet++ para que no
% calcule.
corrientesLineas = zeros(1,16);

end
